simulink model "model"  (R2024b)
settings: Solver=ode45  StartTime=0.0  StopTime=100  RelTol=1e-3
undefined symbols (not defined in the file or in its folder): X, Y, Z
libraries: sm_lib x36, robotlib x19, nesl_utility x9, slpidlib x4, sharedtransform x1
settings Model: Creator=tmood  LastModifiedBy=tmood

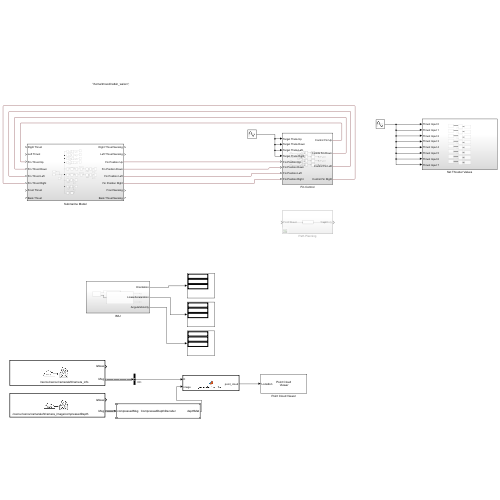
[thumbnail: Simulink's stored preview of the top-level diagram]
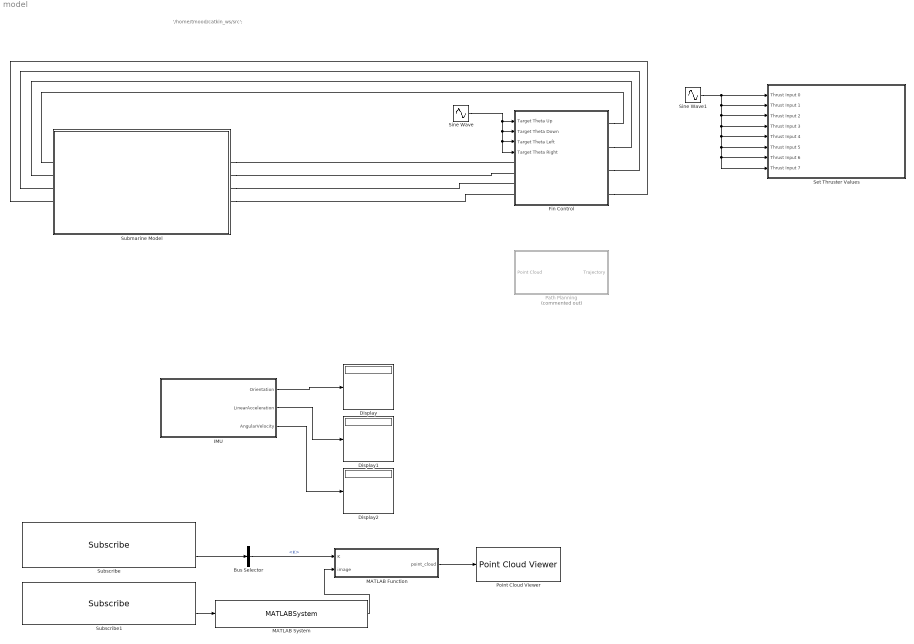
== system model ==
  note: '/home/tmood/catkin_ws/src';
  Bus Selector : BusSelector  OutputSignals=K
  Display : Display
  Display1 : Display
  Display2 : Display
  Fin Control : Subsystem
  IMU : Subsystem
  MATLAB Function : MATLAB Function  TreatAsAtomicUnit=on
  MATLAB System : MATLABSystem  System=CompressedDepthDecoder  SimulateUsing=Interpreted execution
      mask Type: CompressedDepthDecoder
      mask Display:
      | disp('CompressedDepthDecoder');
      | port_label('input',1,'compressedMsg');
      | port_label('output',1,'depthMat');
  Path Planning : Subsystem  Commented=on
  Point Cloud Viewer : PointCloudViewer  FigPos=[665.8 703.6 409.6 300]
  Set Thruster Values : Subsystem
  Sine Wave : Sin  Amplitude=pi/2  SampleTime=0
  Sine Wave1 : Sin  Amplitude=2000  Frequency=0.1  SampleTime=0
  Submarine Model : Subsystem
  Subscribe : robotlib/Subscribe  topicSource=Select from ROS network  topic=/rexrov/rexrov/cameraleft/camera_info  messageType=sensor_msgs/CameraInfo  SampleTime=-1  legacyBusStruct=off  messageQueueLength=1
  Subscribe1 : robotlib/Subscribe  topicSource=Select from ROS network  topic=/rexrov/rexrov/cameraleft/camera_image/compressedDepth  messageType=sensor_msgs/CompressedImage  SampleTime=-1  legacyBusStruct=off  messageQueueLength=1
  wires:
  Sine Wave/1 -> Fin Control/4(Target Theta Right), Fin Control/3(Target Theta Left), Fin Control/2(Target Theta Down), Fin Control/1(Target Theta Up)
  Sine Wave1/1 -> Set Thruster Values/8(Thrust Input 7), Set Thruster Values/7(Thrust Input 6), Set Thruster Values/6(Thrust Input 5), Set Thruster Values/5(Thrust Input 4), Set Thruster Values/4(Thrust Input 3), Set Thruster Values/3(Thrust Input 2), Set Thruster Values/2(Thrust Input 1), Set Thruster Values/1(Thrust Input 0)
  IMU/1(Orientation) -> Display/1
  IMU/2(LinearAcceleration) -> Display1/1
  IMU/3(AngularVelocity) -> Display2/1
  Subscribe/2 -> Bus Selector/1
  Subscribe1/2 -> MATLAB System/1
  MATLAB Function/1(point_cloud) -> Point Cloud Viewer/1
  Bus Selector/1 -> MATLAB Function/1(K)  "<K>"
  MATLAB System/1 -> MATLAB Function/2(image)
  connections:
  Submarine Model/RConn3 -- Fin Control/LConn1
  Submarine Model/RConn4 -- Fin Control/LConn2
  Submarine Model/RConn5 -- Fin Control/LConn3
  Submarine Model/RConn6 -- Fin Control/LConn4
  Fin Control/RConn1 -- Submarine Model/LConn3
  Fin Control/RConn2 -- Submarine Model/LConn4
  Fin Control/RConn3 -- Submarine Model/LConn5
  Fin Control/RConn4 -- Submarine Model/LConn6

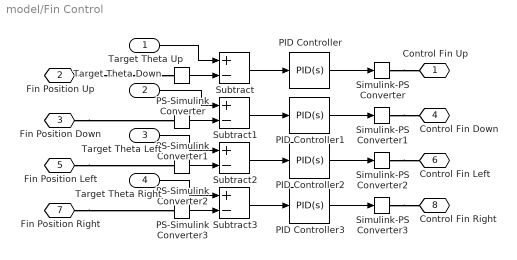
== system model/Fin Control ==
  Target Theta Up : Inport
  Target Theta Down : Inport  Port=2
  Target Theta Left : Inport  Port=3
  Target Theta Right : Inport  Port=4
  PID Controller{,1..3} (4 alike) : slpidlib/PID Controller  Controller=PID  Form=Parallel  TimeDomain=Continuous-time  UseExternalTs=off  SampleTime=-1  IntegratorMethod=Forward Euler  FilterMethod=Forward Euler  ControllerParametersSource=internal  P=1.4  I=0.5  UseKiTs=off  D=1.4  UseExternalDerivativeSource=off  N=100  UseFilter=on  TunerSelectOption=Transfer Function Based (PID Tuner App)  InitialConditionSource=internal  InitialConditionForIntegrator=0.1  InitialConditionForFilter=0  DifferentiatorICPrevScaledInput=0  ExternalReset=none  TrackingMode=off  Kt=1  LimitOutput=off  SatLimitsSource=internal  UpperSaturationLimit=inf  LowerSaturationLimit=-inf  LinearizeAsGain=on  AntiWindupMode=none  Kb=1  LimitIntegrator=off  UpperIntegratorSaturationLimit=inf  LowerIntegratorSaturationLimit=-inf  POutMin=[]  POutMax=[]  IOutMin=[]  IOutMax=[]  DOutMin=[]  DOutMax=[]  NOutMin=[]  NOutMax=[]  SumOutMin=[]  SumOutMax=[]  SaturationOutMin=[]  SaturationOutMax=[]  PParamMin=[]  PParamMax=[]  IParamMin=[]  IParamMax=[]  DParamMin=[]  DParamMax=[]  NParamMin=[]  NParamMax=[]  KbParamMin=[]  KbParamMax=[]  KtParamMin=[]  KtParamMax=[]  KbOutMin=[]  KbOutMax=[]  KtOutMin=[]  KtOutMax=[]  IntegratorOutMin=[]  IntegratorOutMax=[]  FilterOutMin=[]  FilterOutMax=[]  SumI1OutMin=[]  SumI1OutMax=[]  SumI2OutMin=[]  SumI2OutMax=[]  SumI3OutMin=[]  SumI3OutMax=[]  SumI4OutMin=[]  SumI4OutMax=[]  SumDOutMin=[]  SumDOutMax=[]  DifferentiatorOutMin=[]  DifferentiatorOutMax=[]  FilterDiffOutCoefMin=[]  FilterDiffOutCoefMax=[]  ReciprocalOutMin=[]  ReciprocalOutMax=[]  SumDenOutMin=[]  SumDenOutMax=[]  SumNumOutMin=[]  SumNumOutMax=[]  DivideOutMin=[]  DivideOutMax=[]  UdiffTsProdOutMin=[]  UdiffTsProdOutMax=[]  NTsProdOutMin=[]  NTsProdOutMax=[]  UintegralTsProdOutMin=[]  UintegralTsProdOutMax=[]  UngainTsProdOutMin=[]  UngainTsProdOutMax=[]  ClampingZeroOutDataTypeStr=Inherit: Inherit via back propagation  ClampingZeroOutMin=[]  ClampingZeroOutMax=[]  FilterDenConstantOutDataTypeStr=Inherit: Inherit via back propagation  FilterDenConstantOutMin=[]  FilterDenConstantOutMax=[]  PCopyOutDataTypeStr=Inherit: Inherit via back propagation  PCopyOutMin=[]  PCopyOutMax=[]  NCopyOutDataTypeStr=Inherit: Inherit via back propagation  NCopyOutMin=[]  NCopyOutMax=[]  IntegratorContinuousStateAttributes=''  IntegratorStateMustResolveToSignalObject=off  IntegratorRTWStateStorageClass=Auto  FilterContinuousStateAttributes=''  FilterStateMustResolveToSignalObject=off  FilterRTWStateStorageClass=Auto  ParallelPVariant=InternalParameters  IdealPVariant=Disabled  IVariant=InternalParameters  DVariant=InternalParameters  IntegratorVariant=Continuous  SatVariant=Disabled  AWVariant=Passthrough  PCopyVariant=Disabled  TRVariant=Disabled  FdbkBlocksVariant=Forward  IdealPFdbkVariant=Disabled  SatFdbkVariant=Disabled  DerivativeFilterVariant=ContFilter  NVariant=InternalParameters  NCopyVariant=Disabled  FilterICVariant=InternalICsFilter  IntegratorICVariant=InternalICs  ExternalResetVariant=Disabled  TRSumVariant=Passthrough  SumFdbkVariant=Disabled  SumVariant=Sum_PID  TsampFilterVariant=InternalTs  TsampNgainVariant=Passthrough  TsampIntegralVariant=Disabled_SignalSpec  ExternalSaturationOutDataTypeStr=Inherit: Same as second input  DerivativeSourceVariant=ErrorSignal  PreIntVariant=InternalPreInt
  PS-Simulink Converter{,1..3} (4 alike) : nesl_utility/PS-Simulink Converter  PhysicalDomain=network_engine_domain  SubClassName=ps_output  LeftPortType=input  RightPortType=output  PseudoPeriodic=off  Frequencies=[]  VectorFormat=inherit  Unit=inherit  AffineConversion=off
  Simulink-PS Converter{,1..3} (4 alike) : nesl_utility/Simulink-PS Converter  PhysicalDomain=network_engine_domain  SubClassName=ps_input  LeftPortType=input  RightPortType=output  PseudoPeriodic=off  Frequencies=[]  NoiseDistribution=none  NoiseParameters=[]  Unit=1  AffineConversion=off  FilteringAndDerivatives=provide  SimscapeFilterOrder=1  InputFilterTimeConstant=0.001  UdotUserProvided=0
  Subtract{,1..3} (4 alike) : Sum  Inputs=+-
  Control Fin Up : PMIOPort  Side=Right
  Fin Position Up : PMIOPort  Port=2  Side=Left
  Fin Position Down : PMIOPort  Port=3  Side=Left
  Control Fin Down : PMIOPort  Port=4  Side=Right
  Fin Position Left : PMIOPort  Port=5  Side=Left
  Control Fin Left : PMIOPort  Port=6  Side=Right
  Fin Position Right : PMIOPort  Port=7  Side=Left
  Control Fin Right : PMIOPort  Port=8  Side=Right
  wires:
  PID Controller1/1 -> Simulink-PS Converter1/1
  PS-Simulink Converter2/1 -> Subtract2/2
  Target Theta Up/1 -> Subtract/1
  PID Controller2/1 -> Simulink-PS Converter2/1
  PS-Simulink Converter3/1 -> Subtract3/2
  PID Controller/1 -> Simulink-PS Converter/1
  PID Controller3/1 -> Simulink-PS Converter3/1
  Subtract1/1 -> PID Controller1/1
  PS-Simulink Converter1/1 -> Subtract1/2
  Target Theta Down/1 -> Subtract1/1
  PS-Simulink Converter/1 -> Subtract/2
  Target Theta Right/1 -> Subtract3/1
  Subtract/1 -> PID Controller/1
  Subtract2/1 -> PID Controller2/1
  Subtract3/1 -> PID Controller3/1
  Target Theta Left/1 -> Subtract2/1
  connections:
  Fin Position Down/RConn1 -- PS-Simulink Converter1/LConn1
  Simulink-PS Converter2/RConn1 -- Control Fin Left/RConn1
  Simulink-PS Converter/RConn1 -- Control Fin Up/RConn1
  Fin Position Left/RConn1 -- PS-Simulink Converter2/LConn1
  Simulink-PS Converter1/RConn1 -- Control Fin Down/RConn1
  Fin Position Right/RConn1 -- PS-Simulink Converter3/LConn1
  Fin Position Up/RConn1 -- PS-Simulink Converter/LConn1
  Simulink-PS Converter3/RConn1 -- Control Fin Right/RConn1

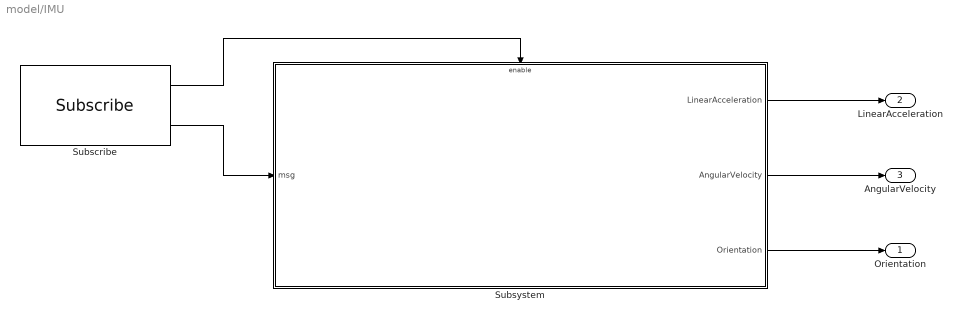
== system model/IMU ==
  Subscribe : robotlib/Subscribe  topicSource=Select from ROS network  topic=/rexrov/imu  messageType=sensor_msgs/Imu  SampleTime=-1  legacyBusStruct=off  messageQueueLength=1
  Subsystem : Subsystem
  Orientation : Outport
  LinearAcceleration : Outport  Port=2
  AngularVelocity : Outport  Port=3
  wires:
  Subscribe/2 -> Subsystem/1(msg)
  Subsystem/1(LinearAcceleration) -> LinearAcceleration/1
  Subsystem/2(AngularVelocity) -> AngularVelocity/1
  Subsystem/3(Orientation) -> Orientation/1
  Subscribe/1 -> Subsystem/Enable

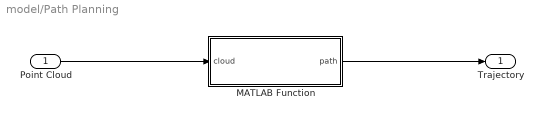
== system model/Path Planning ==
  Point Cloud : Inport
  MATLAB Function : MATLAB Function  TreatAsAtomicUnit=on
  Trajectory : Outport
  wires:
  Point Cloud/1 -> MATLAB Function/1(cloud)
  MATLAB Function/1(path) -> Trajectory/1

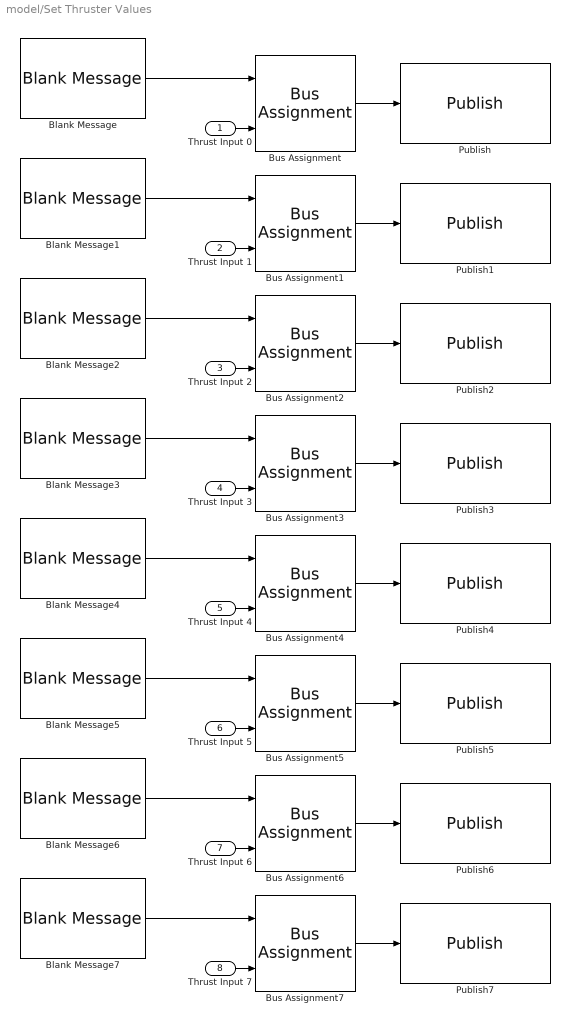
== system model/Set Thruster Values ==
  Thrust Input 0 : Inport
  Thrust Input 1 : Inport  Port=2
  Thrust Input 2 : Inport  Port=3
  Thrust Input 3 : Inport  Port=4
  Thrust Input 4 : Inport  Port=5
  Thrust Input 5 : Inport  Port=6
  Thrust Input 6 : Inport  Port=7
  Thrust Input 7 : Inport  Port=8
  Blank Message{,1..7} (8 alike) : robotlib/Blank Message  messageClass=Message  entityType=uuv_gazebo_ros_plugins_msgs/FloatStamped  messageType=uuv_gazebo_ros_plugins_msgs/FloatStamped  SampleTime=inf  legacyBusStruct=off
  Bus Assignment{,1..7} (8 alike) : BusAssignment  AssignedSignals=Data
  Publish : robotlib/Publish  topicSource=Select from ROS network  topic=/rexrov/thrusters/0/input  messageType=uuv_gazebo_ros_plugins_msgs/FloatStamped  legacyBusStruct=off  messageQueueLength=1
  Publish1 : robotlib/Publish  topicSource=Select from ROS network  topic=/rexrov/thrusters/1/input  messageType=uuv_gazebo_ros_plugins_msgs/FloatStamped  legacyBusStruct=off  messageQueueLength=1
  Publish2 : robotlib/Publish  topicSource=Select from ROS network  topic=/rexrov/thrusters/2/input  messageType=uuv_gazebo_ros_plugins_msgs/FloatStamped  legacyBusStruct=off  messageQueueLength=1
  Publish3 : robotlib/Publish  topicSource=Select from ROS network  topic=/rexrov/thrusters/3/input  messageType=uuv_gazebo_ros_plugins_msgs/FloatStamped  legacyBusStruct=off  messageQueueLength=1
  Publish4 : robotlib/Publish  topicSource=Select from ROS network  topic=/rexrov/thrusters/4/input  messageType=uuv_gazebo_ros_plugins_msgs/FloatStamped  legacyBusStruct=off  messageQueueLength=1
  Publish5 : robotlib/Publish  topicSource=Select from ROS network  topic=/rexrov/thrusters/5/input  messageType=uuv_gazebo_ros_plugins_msgs/FloatStamped  legacyBusStruct=off  messageQueueLength=1
  Publish6 : robotlib/Publish  topicSource=Select from ROS network  topic=/rexrov/thrusters/6/input  messageType=uuv_gazebo_ros_plugins_msgs/FloatStamped  legacyBusStruct=off  messageQueueLength=1
  Publish7 : robotlib/Publish  topicSource=Select from ROS network  topic=/rexrov/thrusters/7/input  messageType=uuv_gazebo_ros_plugins_msgs/FloatStamped  legacyBusStruct=off  messageQueueLength=1
  wires:
  Bus Assignment2/1 -> Publish2/1
  Blank Message7/1 -> Bus Assignment7/1
  Thrust Input 3/1 -> Bus Assignment3/2
  Blank Message6/1 -> Bus Assignment6/1
  Thrust Input 1/1 -> Bus Assignment1/2
  Bus Assignment6/1 -> Publish6/1
  Bus Assignment5/1 -> Publish5/1
  Bus Assignment4/1 -> Publish4/1
  Thrust Input 0/1 -> Bus Assignment/2
  Bus Assignment3/1 -> Publish3/1
  Blank Message/1 -> Bus Assignment/1
  Blank Message4/1 -> Bus Assignment4/1
  Blank Message1/1 -> Bus Assignment1/1
  Bus Assignment/1 -> Publish/1
  Bus Assignment1/1 -> Publish1/1
  Blank Message5/1 -> Bus Assignment5/1
  Thrust Input 6/1 -> Bus Assignment6/2
  Blank Message3/1 -> Bus Assignment3/1
  Blank Message2/1 -> Bus Assignment2/1
  Bus Assignment7/1 -> Publish7/1
  Thrust Input 4/1 -> Bus Assignment4/2
  Thrust Input 5/1 -> Bus Assignment5/2
  Thrust Input 2/1 -> Bus Assignment2/2
  Thrust Input 7/1 -> Bus Assignment7/2

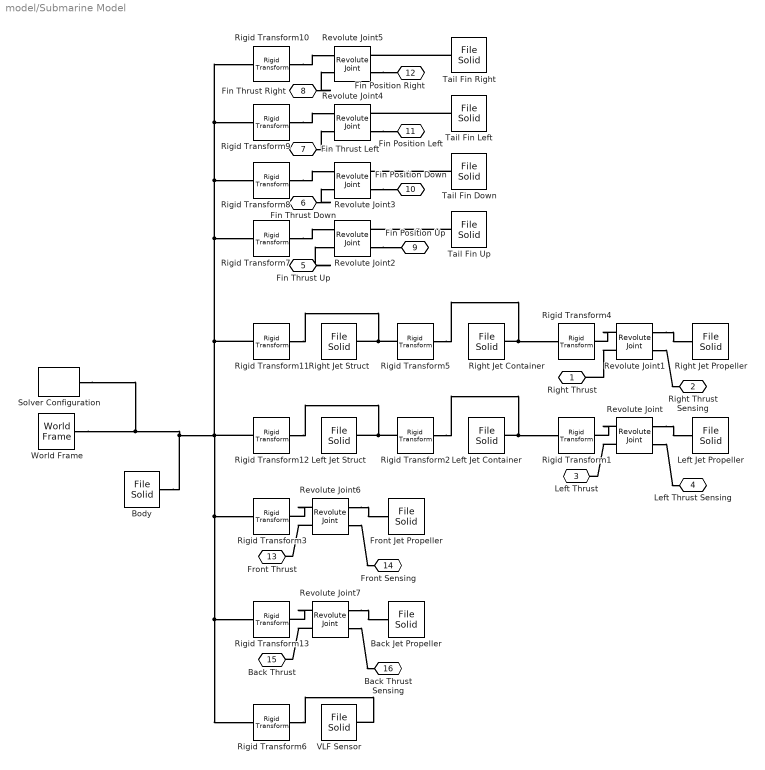
== system model/Submarine Model ==
  Back Jet Propeller : sm_lib/Body Elements/File Solid  ExtGeomFileName=C:\Programming\Competitions\MATLAB\Underwater-Drone\Simulation\Models\jet_turbine.obj  UnitType=Custom  ExtGeomFileUnits=cm  StepReaderType=HEX  ExportConvexHullGeometry=off  InertiaType=CalculateFromGeometry  BasedOnType=Density  Density=DENSITY  DensityUnits=kg/m^3  Mass=1  MassUnits=kg  CenterOfMass=[0 0 0]  CenterOfMassUnits=m  MomentsOfInertia=[1 1 1]  MomentsOfInertiaUnits=kg*m^2  ProductsOfInertia=[0 0 0]  ProductsOfInertiaUnits=kg*m^2  GraphicType=FromGeometry  MarkerShape=Sphere  MarkerSize=10  GraphicVisPropType=SimpleVisualProperties  GraphicDiffuseColor=[0.9 0.9 0.9]  GraphicOpacity=1  GraphicSpecularColor=[0.5 0.5 0.5 1.0]  GraphicAmbientColor=[0.15 0.15 0.15 1.0]  GraphicEmissiveColor=[0.0 0.0 0.0 1.0]  GraphicShininess=75  DoExposeReferenceFrame=on  SerializedFrames=<Frames/>
  Body : sm_lib/Body Elements/File Solid  ExtGeomFileName=C:\Programming\Competitions\MATLAB\Underwater-Drone\Simulation\Models\sub_body.obj  UnitType=Custom  ExtGeomFileUnits=cm  StepReaderType=HEX  ExportConvexHullGeometry=off  InertiaType=CalculateFromGeometry  BasedOnType=Density  Density=DENSITY  DensityUnits=kg/m^3  Mass=1  MassUnits=kg  CenterOfMass=[0 0 0]  CenterOfMassUnits=m  MomentsOfInertia=[1 1 1]  MomentsOfInertiaUnits=kg*m^2  ProductsOfInertia=[0 0 0]  ProductsOfInertiaUnits=kg*m^2  GraphicType=FromGeometry  MarkerShape=Sphere  MarkerSize=10  GraphicVisPropType=SimpleVisualProperties  GraphicDiffuseColor=[0.5 0.5 0.5]  GraphicOpacity=1  GraphicSpecularColor=[0.5 0.5 0.5 1.0]  GraphicAmbientColor=[0.15 0.15 0.15 1.0]  GraphicEmissiveColor=[0.0 0.0 0.0 1.0]  GraphicShininess=75  DoExposeReferenceFrame=on  SerializedFrames=<Frames/>
  Front Jet Propeller : sm_lib/Body Elements/File Solid  ExtGeomFileName=C:\Programming\Competitions\MATLAB\Underwater-Drone\Simulation\Models\jet_turbine.obj  UnitType=Custom  ExtGeomFileUnits=cm  StepReaderType=HEX  ExportConvexHullGeometry=off  InertiaType=CalculateFromGeometry  BasedOnType=Density  Density=DENSITY  DensityUnits=kg/m^3  Mass=1  MassUnits=kg  CenterOfMass=[0 0 0]  CenterOfMassUnits=m  MomentsOfInertia=[1 1 1]  MomentsOfInertiaUnits=kg*m^2  ProductsOfInertia=[0 0 0]  ProductsOfInertiaUnits=kg*m^2  GraphicType=FromGeometry  MarkerShape=Sphere  MarkerSize=10  GraphicVisPropType=SimpleVisualProperties  GraphicDiffuseColor=[0.9 0.9 0.9]  GraphicOpacity=1  GraphicSpecularColor=[0.5 0.5 0.5 1.0]  GraphicAmbientColor=[0.15 0.15 0.15 1.0]  GraphicEmissiveColor=[0.0 0.0 0.0 1.0]  GraphicShininess=75  DoExposeReferenceFrame=on  SerializedFrames=<Frames/>
  Left Jet Container : sm_lib/Body Elements/File Solid  ExtGeomFileName=C:\Programming\Competitions\MATLAB\Underwater-Drone\Simulation\Models\jet_container.obj  UnitType=Custom  ExtGeomFileUnits=mm  StepReaderType=HEX  ExportConvexHullGeometry=off  InertiaType=CalculateFromGeometry  BasedOnType=Density  Density=DENSITY  DensityUnits=kg/m^3  Mass=1  MassUnits=kg  CenterOfMass=[0 0 0]  CenterOfMassUnits=m  MomentsOfInertia=[1 1 1]  MomentsOfInertiaUnits=kg*m^2  ProductsOfInertia=[0 0 0]  ProductsOfInertiaUnits=kg*m^2  GraphicType=FromGeometry  MarkerShape=Sphere  MarkerSize=10  GraphicVisPropType=SimpleVisualProperties  GraphicDiffuseColor=[0.5 0.5 0.5]  GraphicOpacity=1  GraphicSpecularColor=[0.5 0.5 0.5 1.0]  GraphicAmbientColor=[0.15 0.15 0.15 1.0]  GraphicEmissiveColor=[0.0 0.0 0.0 1.0]  GraphicShininess=75  DoExposeReferenceFrame=on  SerializedFrames=<Frames/>
  Left Jet Propeller : sm_lib/Body Elements/File Solid  ExtGeomFileName=C:\Programming\Competitions\MATLAB\Underwater-Drone\Simulation\Models\jet_turbine.obj  UnitType=Custom  ExtGeomFileUnits=cm  StepReaderType=HEX  ExportConvexHullGeometry=off  InertiaType=CalculateFromGeometry  BasedOnType=Density  Density=DENSITY  DensityUnits=kg/m^3  Mass=1  MassUnits=kg  CenterOfMass=[0 0 0]  CenterOfMassUnits=m  MomentsOfInertia=[1 1 1]  MomentsOfInertiaUnits=kg*m^2  ProductsOfInertia=[0 0 0]  ProductsOfInertiaUnits=kg*m^2  GraphicType=FromGeometry  MarkerShape=Sphere  MarkerSize=10  GraphicVisPropType=SimpleVisualProperties  GraphicDiffuseColor=[0.9 0.9 0.9]  GraphicOpacity=1  GraphicSpecularColor=[0.5 0.5 0.5 1.0]  GraphicAmbientColor=[0.15 0.15 0.15 1.0]  GraphicEmissiveColor=[0.0 0.0 0.0 1.0]  GraphicShininess=75  DoExposeReferenceFrame=on  SerializedFrames=<Frames/>
  Left Jet Struct : sm_lib/Body Elements/File Solid  ExtGeomFileName=C:\Programming\Competitions\MATLAB\Underwater-Drone\Simulation\Models\jet_struct.obj  UnitType=Custom  ExtGeomFileUnits=mm  StepReaderType=HEX  ExportConvexHullGeometry=off  InertiaType=CalculateFromGeometry  BasedOnType=Density  Density=DENSITY  DensityUnits=kg/m^3  Mass=1  MassUnits=kg  CenterOfMass=[0 0 0]  CenterOfMassUnits=m  MomentsOfInertia=[1 1 1]  MomentsOfInertiaUnits=kg*m^2  ProductsOfInertia=[0 0 0]  ProductsOfInertiaUnits=kg*m^2  GraphicType=FromGeometry  MarkerShape=Sphere  MarkerSize=10  GraphicVisPropType=SimpleVisualProperties  GraphicDiffuseColor=[0.5 0.5 0.5]  GraphicOpacity=1  GraphicSpecularColor=[0.5 0.5 0.5 1.0]  GraphicAmbientColor=[0.15 0.15 0.15 1.0]  GraphicEmissiveColor=[0.0 0.0 0.0 1.0]  GraphicShininess=75  DoExposeReferenceFrame=on  SerializedFrames=<Frames/>
  Revolute Joint{,1,6..7} (4 alike) : sm_lib/Joints/Revolute Joint  JointMode=Normal  CompositeWrenchDir=FollowerOnBase  CompositeWrenchFrame=BaseFrame  SenseConstraintForce=off  SenseConstraintTorque=off  SenseTotalForce=off  SenseTotalTorque=off  PositionTargetSpecify=off  PositionTargetPriority=High  PositionTargetValue=0  PositionTargetValueUnits=deg  VelocityTargetSpecify=off  VelocityTargetPriority=High  VelocityTargetValue=0  VelocityTargetValueUnits=deg/s  EquilibriumPosition=0  EquilibriumPositionUnits=deg  SpringStiffness=0  SpringStiffnessUnits=N*m/deg  DampingCoefficient=0  DampingCoefficientUnits=N*m/(deg/s)  LowerLimitSpecify=off  LowerLimitBound=-90  LowerLimitBoundUnits=deg  LowerLimitStiffness=1e4  LowerLimitStiffnessUnits=N*m/deg  LowerLimitDamping=10  LowerLimitDampingUnits=N*m/(deg/s)  LowerLimitTransitionRegionWidth=0.1  LowerLimitTransitionRegionWidthUnits=deg  UpperLimitSpecify=off  UpperLimitBound=90  UpperLimitBoundUnits=deg  UpperLimitStiffness=1e4  UpperLimitStiffnessUnits=N*m/deg  UpperLimitDamping=10  UpperLimitDampingUnits=N*m/(deg/s)  UpperLimitTransitionRegionWidth=0.1  UpperLimitTransitionRegionWidthUnits=deg  TorqueActuationMode=InputTorque  MotionActuationMode=ComputedMotion  SensePosition=off  SenseVelocity=off  SenseAcceleration=off  SenseTorqueForce=on  SenseLowerLimitTorqueForce=off  SenseUpperLimitTorqueForce=off
  Revolute Joint{2..5} (4 alike) : sm_lib/Joints/Revolute Joint  JointMode=Normal  CompositeWrenchDir=FollowerOnBase  CompositeWrenchFrame=BaseFrame  SenseConstraintForce=off  SenseConstraintTorque=off  SenseTotalForce=off  SenseTotalTorque=off  PositionTargetSpecify=off  PositionTargetPriority=High  PositionTargetValue=0  PositionTargetValueUnits=deg  VelocityTargetSpecify=off  VelocityTargetPriority=High  VelocityTargetValue=0  VelocityTargetValueUnits=deg/s  EquilibriumPosition=0  EquilibriumPositionUnits=deg  SpringStiffness=0  SpringStiffnessUnits=N*m/deg  DampingCoefficient=0  DampingCoefficientUnits=N*m/(deg/s)  LowerLimitSpecify=off  LowerLimitBound=-90  LowerLimitBoundUnits=deg  LowerLimitStiffness=1e4  LowerLimitStiffnessUnits=N*m/deg  LowerLimitDamping=10  LowerLimitDampingUnits=N*m/(deg/s)  LowerLimitTransitionRegionWidth=0.1  LowerLimitTransitionRegionWidthUnits=deg  UpperLimitSpecify=off  UpperLimitBound=90  UpperLimitBoundUnits=deg  UpperLimitStiffness=1e4  UpperLimitStiffnessUnits=N*m/deg  UpperLimitDamping=10  UpperLimitDampingUnits=N*m/(deg/s)  UpperLimitTransitionRegionWidth=0.1  UpperLimitTransitionRegionWidthUnits=deg  TorqueActuationMode=InputTorque  MotionActuationMode=ComputedMotion  SensePosition=on  SenseVelocity=off  SenseAcceleration=off  SenseTorqueForce=off  SenseLowerLimitTorqueForce=off  SenseUpperLimitTorqueForce=off
  Right Jet Container : sm_lib/Body Elements/File Solid  ExtGeomFileName=C:\Programming\Competitions\MATLAB\Underwater-Drone\Simulation\Models\jet_container.obj  UnitType=Custom  ExtGeomFileUnits=mm  StepReaderType=HEX  ExportConvexHullGeometry=off  InertiaType=CalculateFromGeometry  BasedOnType=Density  Density=DENSITY  DensityUnits=kg/m^3  Mass=1  MassUnits=kg  CenterOfMass=[0 0 0]  CenterOfMassUnits=m  MomentsOfInertia=[1 1 1]  MomentsOfInertiaUnits=kg*m^2  ProductsOfInertia=[0 0 0]  ProductsOfInertiaUnits=kg*m^2  GraphicType=FromGeometry  MarkerShape=Sphere  MarkerSize=10  GraphicVisPropType=SimpleVisualProperties  GraphicDiffuseColor=[0.5 0.5 0.5]  GraphicOpacity=1  GraphicSpecularColor=[0.5 0.5 0.5 1.0]  GraphicAmbientColor=[0.15 0.15 0.15 1.0]  GraphicEmissiveColor=[0.0 0.0 0.0 1.0]  GraphicShininess=75  DoExposeReferenceFrame=on  SerializedFrames=<Frames/>
  Right Jet Propeller : sm_lib/Body Elements/File Solid  ExtGeomFileName=C:\Programming\Competitions\MATLAB\Underwater-Drone\Simulation\Models\jet_turbine.obj  UnitType=Custom  ExtGeomFileUnits=cm  StepReaderType=HEX  ExportConvexHullGeometry=off  InertiaType=CalculateFromGeometry  BasedOnType=Density  Density=DENSITY  DensityUnits=kg/m^3  Mass=1  MassUnits=kg  CenterOfMass=[0 0 0]  CenterOfMassUnits=m  MomentsOfInertia=[1 1 1]  MomentsOfInertiaUnits=kg*m^2  ProductsOfInertia=[0 0 0]  ProductsOfInertiaUnits=kg*m^2  GraphicType=FromGeometry  MarkerShape=Sphere  MarkerSize=10  GraphicVisPropType=SimpleVisualProperties  GraphicDiffuseColor=[0.9 0.9 0.9]  GraphicOpacity=1  GraphicSpecularColor=[0.5 0.5 0.5 1.0]  GraphicAmbientColor=[0.15 0.15 0.15 1.0]  GraphicEmissiveColor=[0.0 0.0 0.0 1.0]  GraphicShininess=75  DoExposeReferenceFrame=on  SerializedFrames=<Frames/>
  Right Jet Struct : sm_lib/Body Elements/File Solid  ExtGeomFileName=C:\Programming\Competitions\MATLAB\Underwater-Drone\Simulation\Models\jet_struct.obj  UnitType=Custom  ExtGeomFileUnits=mm  StepReaderType=HEX  ExportConvexHullGeometry=off  InertiaType=CalculateFromGeometry  BasedOnType=Density  Density=DENSITY  DensityUnits=kg/m^3  Mass=1  MassUnits=kg  CenterOfMass=[0 0 0]  CenterOfMassUnits=m  MomentsOfInertia=[1 1 1]  MomentsOfInertiaUnits=kg*m^2  ProductsOfInertia=[0 0 0]  ProductsOfInertiaUnits=kg*m^2  GraphicType=FromGeometry  MarkerShape=Sphere  MarkerSize=10  GraphicVisPropType=SimpleVisualProperties  GraphicDiffuseColor=[0.5 0.5 0.5]  GraphicOpacity=1  GraphicSpecularColor=[0.5 0.5 0.5 1.0]  GraphicAmbientColor=[0.15 0.15 0.15 1.0]  GraphicEmissiveColor=[0.0 0.0 0.0 1.0]  GraphicShininess=75  DoExposeReferenceFrame=on  SerializedFrames=<Frames/>
  Rigid Transform1 : sm_lib/Frames and Transforms/Rigid Transform  RotationMethod=RotationSequence  FollAlignAxisA=+X  BaseAlignAxisA=+Y  FollAlignAxisB=+Y  BaseAlignAxisB=+Z  RotationStandardAxis=+Z  RotationAngle=0  RotationAngleUnits=deg  RotationArbitraryAxis=[0 0 1]  RotationSequenceAxes=BaseAxes  RotationSequence=XYZ  RotationSequenceAngles=[-90 0 0]  RotationSequenceAnglesUnits=deg  RotationMatrix=[1 0 0;0 1 0;0 0 1]  Quaternion=[1 0 0 0]  TranslationMethod=Cartesian  TranslationCartesianOffset=[0 0.85 0]  TranslationCartesianOffsetUnits=m  TranslationStandardAxis=+Z  TranslationStandardOffset=0  TranslationStandardOffsetUnits=m  TranslationROffset=0  TranslationROffsetUnits=m  TranslationThetaOffset=0  TranslationThetaOffsetUnits=deg  TranslationZOffset=0  TranslationZOffsetUnits=m
  Rigid Transform10 : sm_lib/Frames and Transforms/Rigid Transform  RotationMethod=RotationSequence  FollAlignAxisA=+X  BaseAlignAxisA=+Y  FollAlignAxisB=+Y  BaseAlignAxisB=+Z  RotationStandardAxis=+Z  RotationAngle=90  RotationAngleUnits=deg  RotationArbitraryAxis=[0 0 1]  RotationSequenceAxes=BaseAxes  RotationSequence=XYZ  RotationSequenceAngles=[-90 0 0]  RotationSequenceAnglesUnits=deg  RotationMatrix=[1 0 0;0 1 0;0 0 1]  Quaternion=[1 0 0 0]  TranslationMethod=Cartesian  TranslationCartesianOffset=[1.8 0.35 0]  TranslationCartesianOffsetUnits=m  TranslationStandardAxis=+Y  TranslationStandardOffset=100  TranslationStandardOffsetUnits=m  TranslationROffset=0  TranslationROffsetUnits=m  TranslationThetaOffset=0  TranslationThetaOffsetUnits=deg  TranslationZOffset=0  TranslationZOffsetUnits=m
  Rigid Transform11 : sm_lib/Frames and Transforms/Rigid Transform  RotationMethod=RotationSequence  FollAlignAxisA=+X  BaseAlignAxisA=+Y  FollAlignAxisB=+Y  BaseAlignAxisB=+Z  RotationStandardAxis=+Z  RotationAngle=0  RotationAngleUnits=deg  RotationArbitraryAxis=[0 0 1]  RotationSequenceAxes=BaseAxes  RotationSequence=XYZ  RotationSequenceAngles=[0 0 90]  RotationSequenceAnglesUnits=deg  RotationMatrix=[1 0 0;0 1 0;0 0 1]  Quaternion=[1 0 0 0]  TranslationMethod=Cartesian  TranslationCartesianOffset=[1.5 0.7 0]  TranslationCartesianOffsetUnits=m  TranslationStandardAxis=+Z  TranslationStandardOffset=0  TranslationStandardOffsetUnits=m  TranslationROffset=0  TranslationROffsetUnits=m  TranslationThetaOffset=0  TranslationThetaOffsetUnits=deg  TranslationZOffset=0  TranslationZOffsetUnits=m
  Rigid Transform12 : sm_lib/Frames and Transforms/Rigid Transform  RotationMethod=RotationSequence  FollAlignAxisA=+X  BaseAlignAxisA=+Y  FollAlignAxisB=+Y  BaseAlignAxisB=+Z  RotationStandardAxis=+Z  RotationAngle=90  RotationAngleUnits=deg  RotationArbitraryAxis=[0 0 1]  RotationSequenceAxes=BaseAxes  RotationSequence=XYZ  RotationSequenceAngles=[0 180 90]  RotationSequenceAnglesUnits=deg  RotationMatrix=[1 0 0;0 1 0;0 0 1]  Quaternion=[1 0 0 0]  TranslationMethod=Cartesian  TranslationCartesianOffset=[1.5 -0.7 0]  TranslationCartesianOffsetUnits=m  TranslationStandardAxis=+Y  TranslationStandardOffset=100  TranslationStandardOffsetUnits=m  TranslationROffset=0  TranslationROffsetUnits=m  TranslationThetaOffset=0  TranslationThetaOffsetUnits=deg  TranslationZOffset=0  TranslationZOffsetUnits=m
  Rigid Transform13 : sm_lib/Frames and Transforms/Rigid Transform  RotationMethod=RotationSequence  FollAlignAxisA=+X  BaseAlignAxisA=+Y  FollAlignAxisB=+Y  BaseAlignAxisB=+Z  RotationStandardAxis=+Z  RotationAngle=0  RotationAngleUnits=deg  RotationArbitraryAxis=[0 0 1]  RotationSequenceAxes=BaseAxes  RotationSequence=XYZ  RotationSequenceAngles=[0 0 0]  RotationSequenceAnglesUnits=deg  RotationMatrix=[1 0 0;0 1 0;0 0 1]  Quaternion=[1 0 0 0]  TranslationMethod=Cartesian  TranslationCartesianOffset=[1.2 0 0.35]  TranslationCartesianOffsetUnits=m  TranslationStandardAxis=+Z  TranslationStandardOffset=0  TranslationStandardOffsetUnits=m  TranslationROffset=0  TranslationROffsetUnits=m  TranslationThetaOffset=0  TranslationThetaOffsetUnits=deg  TranslationZOffset=0  TranslationZOffsetUnits=m
  Rigid Transform2 : sm_lib/Frames and Transforms/Rigid Transform  RotationMethod=None  FollAlignAxisA=+X  BaseAlignAxisA=+Y  FollAlignAxisB=+Y  BaseAlignAxisB=+Z  RotationStandardAxis=+Z  RotationAngle=0  RotationAngleUnits=deg  RotationArbitraryAxis=[0 0 1]  RotationSequenceAxes=FollowerAxes  RotationSequence=XYX  RotationSequenceAngles=[0 0 0]  RotationSequenceAnglesUnits=deg  RotationMatrix=[1 0 0;0 1 0;0 0 1]  Quaternion=[1 0 0 0]  TranslationMethod=None  TranslationCartesianOffset=[0 0 0]  TranslationCartesianOffsetUnits=m  TranslationStandardAxis=+Z  TranslationStandardOffset=0  TranslationStandardOffsetUnits=m  TranslationROffset=0  TranslationROffsetUnits=m  TranslationThetaOffset=0  TranslationThetaOffsetUnits=deg  TranslationZOffset=0  TranslationZOffsetUnits=m
  Rigid Transform3 : sm_lib/Frames and Transforms/Rigid Transform  RotationMethod=RotationSequence  FollAlignAxisA=+X  BaseAlignAxisA=+Y  FollAlignAxisB=+Y  BaseAlignAxisB=+Z  RotationStandardAxis=+Z  RotationAngle=0  RotationAngleUnits=deg  RotationArbitraryAxis=[0 0 1]  RotationSequenceAxes=BaseAxes  RotationSequence=XYZ  RotationSequenceAngles=[0 0 0]  RotationSequenceAnglesUnits=deg  RotationMatrix=[1 0 0;0 1 0;0 0 1]  Quaternion=[1 0 0 0]  TranslationMethod=Cartesian  TranslationCartesianOffset=[0.5 0 0.35]  TranslationCartesianOffsetUnits=m  TranslationStandardAxis=+Z  TranslationStandardOffset=0  TranslationStandardOffsetUnits=m  TranslationROffset=0  TranslationROffsetUnits=m  TranslationThetaOffset=0  TranslationThetaOffsetUnits=deg  TranslationZOffset=0  TranslationZOffsetUnits=m
  Rigid Transform4 : sm_lib/Frames and Transforms/Rigid Transform  RotationMethod=RotationSequence  FollAlignAxisA=+X  BaseAlignAxisA=+Y  FollAlignAxisB=+Y  BaseAlignAxisB=+Z  RotationStandardAxis=+Z  RotationAngle=0  RotationAngleUnits=deg  RotationArbitraryAxis=[0 0 1]  RotationSequenceAxes=FollowerAxes  RotationSequence=XYZ  RotationSequenceAngles=[-90 0 0]  RotationSequenceAnglesUnits=deg  RotationMatrix=[1 0 0;0 1 0;0 0 1]  Quaternion=[1 0 0 0]  TranslationMethod=Cartesian  TranslationCartesianOffset=[0 0.85 0]  TranslationCartesianOffsetUnits=m  TranslationStandardAxis=+Z  TranslationStandardOffset=0  TranslationStandardOffsetUnits=m  TranslationROffset=0  TranslationROffsetUnits=m  TranslationThetaOffset=0  TranslationThetaOffsetUnits=deg  TranslationZOffset=0  TranslationZOffsetUnits=m
  Rigid Transform5 : sm_lib/Frames and Transforms/Rigid Transform  RotationMethod=None  FollAlignAxisA=+X  BaseAlignAxisA=+Y  FollAlignAxisB=+Y  BaseAlignAxisB=+Z  RotationStandardAxis=+Z  RotationAngle=0  RotationAngleUnits=deg  RotationArbitraryAxis=[0 0 1]  RotationSequenceAxes=FollowerAxes  RotationSequence=XYX  RotationSequenceAngles=[0 0 0]  RotationSequenceAnglesUnits=deg  RotationMatrix=[1 0 0;0 1 0;0 0 1]  Quaternion=[1 0 0 0]  TranslationMethod=None  TranslationCartesianOffset=[0 0 0]  TranslationCartesianOffsetUnits=m  TranslationStandardAxis=+Z  TranslationStandardOffset=0  TranslationStandardOffsetUnits=m  TranslationROffset=0  TranslationROffsetUnits=m  TranslationThetaOffset=0  TranslationThetaOffsetUnits=deg  TranslationZOffset=0  TranslationZOffsetUnits=m
  Rigid Transform6 : sm_lib/Frames and Transforms/Rigid Transform  RotationMethod=RotationSequence  FollAlignAxisA=+X  BaseAlignAxisA=+Y  FollAlignAxisB=+Y  BaseAlignAxisB=+Z  RotationStandardAxis=+Z  RotationAngle=0  RotationAngleUnits=deg  RotationArbitraryAxis=[0 0 1]  RotationSequenceAxes=BaseAxes  RotationSequence=XYZ  RotationSequenceAngles=[0 90 0]  RotationSequenceAnglesUnits=deg  RotationMatrix=[1 0 0;0 1 0;0 0 1]  Quaternion=[1 0 0 0]  TranslationMethod=Cartesian  TranslationCartesianOffset=[-0.05 0 0]  TranslationCartesianOffsetUnits=m  TranslationStandardAxis=+Z  TranslationStandardOffset=0  TranslationStandardOffsetUnits=m  TranslationROffset=0  TranslationROffsetUnits=m  TranslationThetaOffset=0  TranslationThetaOffsetUnits=deg  TranslationZOffset=0  TranslationZOffsetUnits=m
  Rigid Transform7 : sm_lib/Frames and Transforms/Rigid Transform  RotationMethod=RotationSequence  FollAlignAxisA=+X  BaseAlignAxisA=+Y  FollAlignAxisB=+Y  BaseAlignAxisB=+Z  RotationStandardAxis=+Z  RotationAngle=90  RotationAngleUnits=deg  RotationArbitraryAxis=[0 0 1]  RotationSequenceAxes=BaseAxes  RotationSequence=XYZ  RotationSequenceAngles=[0 0 0]  RotationSequenceAnglesUnits=deg  RotationMatrix=[1 0 0;0 1 0;0 0 1]  Quaternion=[1 0 0 0]  TranslationMethod=Cartesian  TranslationCartesianOffset=[1.8 0 0.3]  TranslationCartesianOffsetUnits=m  TranslationStandardAxis=+Y  TranslationStandardOffset=100  TranslationStandardOffsetUnits=m  TranslationROffset=0  TranslationROffsetUnits=m  TranslationThetaOffset=0  TranslationThetaOffsetUnits=deg  TranslationZOffset=0  TranslationZOffsetUnits=m
  Rigid Transform8 : sm_lib/Frames and Transforms/Rigid Transform  RotationMethod=RotationSequence  FollAlignAxisA=+X  BaseAlignAxisA=+Y  FollAlignAxisB=+Y  BaseAlignAxisB=+Z  RotationStandardAxis=+Z  RotationAngle=90  RotationAngleUnits=deg  RotationArbitraryAxis=[0 0 1]  RotationSequenceAxes=BaseAxes  RotationSequence=XYZ  RotationSequenceAngles=[180 0 0]  RotationSequenceAnglesUnits=deg  RotationMatrix=[1 0 0;0 1 0;0 0 1]  Quaternion=[1 0 0 0]  TranslationMethod=Cartesian  TranslationCartesianOffset=[1.8 0 -0.3]  TranslationCartesianOffsetUnits=m  TranslationStandardAxis=+Y  TranslationStandardOffset=100  TranslationStandardOffsetUnits=m  TranslationROffset=0  TranslationROffsetUnits=m  TranslationThetaOffset=0  TranslationThetaOffsetUnits=deg  TranslationZOffset=0  TranslationZOffsetUnits=m
  Rigid Transform9 : sm_lib/Frames and Transforms/Rigid Transform  RotationMethod=RotationSequence  FollAlignAxisA=+X  BaseAlignAxisA=+Y  FollAlignAxisB=+Y  BaseAlignAxisB=+Z  RotationStandardAxis=+Z  RotationAngle=90  RotationAngleUnits=deg  RotationArbitraryAxis=[0 0 1]  RotationSequenceAxes=BaseAxes  RotationSequence=XYZ  RotationSequenceAngles=[90 0 0]  RotationSequenceAnglesUnits=deg  RotationMatrix=[1 0 0;0 1 0;0 0 1]  Quaternion=[1 0 0 0]  TranslationMethod=Cartesian  TranslationCartesianOffset=[1.8 -0.35 0]  TranslationCartesianOffsetUnits=m  TranslationStandardAxis=+Y  TranslationStandardOffset=100  TranslationStandardOffsetUnits=m  TranslationROffset=0  TranslationROffsetUnits=m  TranslationThetaOffset=0  TranslationThetaOffsetUnits=deg  TranslationZOffset=0  TranslationZOffsetUnits=m
  Solver Configuration : nesl_utility/Solver Configuration  PhysicalDomain=network_engine_domain  SubClassName=solver  LeftPortType=input  RightPortType=generic  Tones=[]  Harmonics=[]  SimulateNoise=off  Profile=off  UseLocalSampling=off  EnableSwitchedLinearOptims=on  FrequencyDomain=off  UseCCode=off  RelTol=0.001  AbsTol=0.001  MinStep=1e-09  ToWorkspace=off  RevertToSquareIcSolve=off  NumHomotopyIterations=100  PhasorMode=off  PhasorModeNumHarmonics=1  ConsistencySolver=NEWTON_XTOL_AFTER_FTOL  IndexReductionMethod=DerivativeReplacement  DoDC=off  ResidualTolerance=1e-09  ConsistencyTolSource=GLOBAL  ConsistencyAbsTol=0.001  ConsistencyRelTol=0.001  ConsistencyTolFactor=0.001  UseLocalSolver=off  LocalSolverChoice=NE_BACKWARD_EULER_ADVANCER  ResolveIndetEquations=on  FunctionEvalNumThread=1  LocalSolverSampleTime=0.001  DoFixedCost=off  MaxNonlinIter=3  MaxModeIter=2  ComputeImpulses=off  ImpulseIterations=2  LinearAlgebra=auto  LinearAlgebraNumThread=0  EquationFormulation=NE_TIME_EF  DelaysMemoryBudget=1024  AutomaticFiltering=on  FilteringTimeConstant=0.001  PartitionStorageMethod=AS_NEEDED  PartitionMemoryBudget=1024  PartitionMethod=ROBUST  MultibodyUseLocalSolver=off  MultibodyLocalSolverChoice=ODE1  MultibodyLocalSolverSampleTime=0.001
  Tail Fin Down : sm_lib/Body Elements/File Solid  ExtGeomFileName=C:\Programming\Competitions\MATLAB\Underwater-Drone\Simulation\Models\tail_fin.obj  UnitType=Custom  ExtGeomFileUnits=cm  StepReaderType=HEX  ExportConvexHullGeometry=off  InertiaType=CalculateFromGeometry  BasedOnType=Density  Density=DENSITY  DensityUnits=kg/m^3  Mass=1  MassUnits=kg  CenterOfMass=[0 0 0]  CenterOfMassUnits=m  MomentsOfInertia=[1 1 1]  MomentsOfInertiaUnits=kg*m^2  ProductsOfInertia=[0 0 0]  ProductsOfInertiaUnits=kg*m^2  GraphicType=FromGeometry  MarkerShape=Sphere  MarkerSize=10  GraphicVisPropType=SimpleVisualProperties  GraphicDiffuseColor=[0.5 0.5 0.5]  GraphicOpacity=1  GraphicSpecularColor=[0.5 0.5 0.5 1.0]  GraphicAmbientColor=[0.15 0.15 0.15 1.0]  GraphicEmissiveColor=[0.0 0.0 0.0 1.0]  GraphicShininess=75  DoExposeReferenceFrame=on  SerializedFrames=<Frames/>
  Tail Fin Left : sm_lib/Body Elements/File Solid  ExtGeomFileName=C:\Programming\Competitions\MATLAB\Underwater-Drone\Simulation\Models\tail_fin.obj  UnitType=Custom  ExtGeomFileUnits=cm  StepReaderType=HEX  ExportConvexHullGeometry=off  InertiaType=CalculateFromGeometry  BasedOnType=Density  Density=DENSITY  DensityUnits=kg/m^3  Mass=1  MassUnits=kg  CenterOfMass=[0 0 0]  CenterOfMassUnits=m  MomentsOfInertia=[1 1 1]  MomentsOfInertiaUnits=kg*m^2  ProductsOfInertia=[0 0 0]  ProductsOfInertiaUnits=kg*m^2  GraphicType=FromGeometry  MarkerShape=Sphere  MarkerSize=10  GraphicVisPropType=SimpleVisualProperties  GraphicDiffuseColor=[0.5 0.5 0.5]  GraphicOpacity=1  GraphicSpecularColor=[0.5 0.5 0.5 1.0]  GraphicAmbientColor=[0.15 0.15 0.15 1.0]  GraphicEmissiveColor=[0.0 0.0 0.0 1.0]  GraphicShininess=75  DoExposeReferenceFrame=on  SerializedFrames=<Frames/>
  Tail Fin Right : sm_lib/Body Elements/File Solid  ExtGeomFileName=C:\Programming\Competitions\MATLAB\Underwater-Drone\Simulation\Models\tail_fin.obj  UnitType=Custom  ExtGeomFileUnits=cm  StepReaderType=HEX  ExportConvexHullGeometry=off  InertiaType=CalculateFromGeometry  BasedOnType=Density  Density=DENSITY  DensityUnits=kg/m^3  Mass=1  MassUnits=kg  CenterOfMass=[0 0 0]  CenterOfMassUnits=m  MomentsOfInertia=[1 1 1]  MomentsOfInertiaUnits=kg*m^2  ProductsOfInertia=[0 0 0]  ProductsOfInertiaUnits=kg*m^2  GraphicType=FromGeometry  MarkerShape=Sphere  MarkerSize=10  GraphicVisPropType=SimpleVisualProperties  GraphicDiffuseColor=[0.5 0.5 0.5]  GraphicOpacity=1  GraphicSpecularColor=[0.5 0.5 0.5 1.0]  GraphicAmbientColor=[0.15 0.15 0.15 1.0]  GraphicEmissiveColor=[0.0 0.0 0.0 1.0]  GraphicShininess=75  DoExposeReferenceFrame=on  SerializedFrames=<Frames/>
  Tail Fin Up : sm_lib/Body Elements/File Solid  ExtGeomFileName=C:\Programming\Competitions\MATLAB\Underwater-Drone\Simulation\Models\tail_fin.obj  UnitType=Custom  ExtGeomFileUnits=cm  StepReaderType=HEX  ExportConvexHullGeometry=off  InertiaType=CalculateFromGeometry  BasedOnType=Density  Density=DENSITY  DensityUnits=kg/m^3  Mass=1  MassUnits=kg  CenterOfMass=[0 0 0]  CenterOfMassUnits=m  MomentsOfInertia=[1 1 1]  MomentsOfInertiaUnits=kg*m^2  ProductsOfInertia=[0 0 0]  ProductsOfInertiaUnits=kg*m^2  GraphicType=FromGeometry  MarkerShape=Sphere  MarkerSize=10  GraphicVisPropType=SimpleVisualProperties  GraphicDiffuseColor=[0.5 0.5 0.5]  GraphicOpacity=1  GraphicSpecularColor=[0.5 0.5 0.5 1.0]  GraphicAmbientColor=[0.15 0.15 0.15 1.0]  GraphicEmissiveColor=[0.0 0.0 0.0 1.0]  GraphicShininess=75  DoExposeReferenceFrame=on  SerializedFrames=<Frames/>
  VLF Sensor : sm_lib/Body Elements/File Solid  ExtGeomFileName=C:\Programming\Competitions\MATLAB\Underwater-Drone\Simulation\Models\vlf_distance_sensor.obj  UnitType=Custom  ExtGeomFileUnits=mm  StepReaderType=HEX  ExportConvexHullGeometry=off  InertiaType=CalculateFromGeometry  BasedOnType=Density  Density=DENSITY  DensityUnits=kg/m^3  Mass=1  MassUnits=kg  CenterOfMass=[0 0 0]  CenterOfMassUnits=m  MomentsOfInertia=[1 1 1]  MomentsOfInertiaUnits=kg*m^2  ProductsOfInertia=[0 0 0]  ProductsOfInertiaUnits=kg*m^2  GraphicType=FromGeometry  MarkerShape=Sphere  MarkerSize=10  GraphicVisPropType=SimpleVisualProperties  GraphicDiffuseColor=[0.5 0.5 0.5]  GraphicOpacity=1  GraphicSpecularColor=[0.5 0.5 0.5 1.0]  GraphicAmbientColor=[0.15 0.15 0.15 1.0]  GraphicEmissiveColor=[0.0 0.0 0.0 1.0]  GraphicShininess=75  DoExposeReferenceFrame=on  SerializedFrames=<Frames/>
  World Frame : sm_lib/Frames and Transforms/World Frame
  Right Thrust : PMIOPort  Side=Left
  Right Thrust Sensing : PMIOPort  Port=2  Side=Right
  Left Thrust : PMIOPort  Port=3  Side=Left
  Left Thrust Sensing : PMIOPort  Port=4  Side=Right
  Fin Thrust Up : PMIOPort  Port=5  Side=Left
  Fin Thrust Down : PMIOPort  Port=6  Side=Left
  Fin Thrust Left : PMIOPort  Port=7  Side=Left
  Fin Thrust Right : PMIOPort  Port=8  Side=Left
  Fin Position Up : PMIOPort  Port=9  Side=Right
  Fin Position Down : PMIOPort  Port=10  Side=Right
  Fin Position Left : PMIOPort  Port=11  Side=Right
  Fin Position Right : PMIOPort  Port=12  Side=Right
  Front Thrust : PMIOPort  Port=13  Side=Left
  Front Sensing : PMIOPort  Port=14  Side=Right
  Back Thrust : PMIOPort  Port=15  Side=Left
  Back Thrust Sensing : PMIOPort  Port=16  Side=Right
  connections:
  Rigid Transform2/LConn1 -- Rigid Transform12/RConn1 -- Left Jet Struct/RConn1
  Rigid Transform5/LConn1 -- Rigid Transform11/RConn1 -- Right Jet Struct/RConn1
  World Frame/RConn1 -- Body/RConn1 -- Rigid Transform3/LConn1 -- Rigid Transform13/LConn1 -- Rigid Transform6/LConn1 -- Rigid Transform12/LConn1 -- Rigid Transform11/LConn1 -- Rigid Transform9/LConn1 -- Rigid Transform10/LConn1 -- Rigid Transform8/LConn1 -- Rigid Transform7/LConn1 -- Solver Configuration/RConn1
  Right Jet Container/RConn1 -- Rigid Transform5/RConn1 -- Rigid Transform4/LConn1
  Revolute Joint/LConn1 -- Rigid Transform1/RConn1
  Revolute Joint/RConn1 -- Left Jet Propeller/RConn1
  Revolute Joint1/RConn1 -- Right Jet Propeller/RConn1
  Revolute Joint1/LConn1 -- Rigid Transform4/RConn1
  Rigid Transform2/RConn1 -- Rigid Transform1/LConn1 -- Left Jet Container/RConn1
  Rigid Transform6/RConn1 -- VLF Sensor/RConn1
  Revolute Joint/LConn2 -- Left Thrust/RConn1
  Revolute Joint/RConn2 -- Left Thrust Sensing/RConn1
  Revolute Joint1/RConn2 -- Right Thrust Sensing/RConn1
  Revolute Joint1/LConn2 -- Right Thrust/RConn1
  Rigid Transform7/RConn1 -- Revolute Joint2/LConn1
  Tail Fin Up/RConn1 -- Revolute Joint2/RConn1
  Rigid Transform8/RConn1 -- Revolute Joint3/LConn1
  Tail Fin Down/RConn1 -- Revolute Joint3/RConn1
  Rigid Transform9/RConn1 -- Revolute Joint4/LConn1
  Tail Fin Left/RConn1 -- Revolute Joint4/RConn1
  Rigid Transform10/RConn1 -- Revolute Joint5/LConn1
  Tail Fin Right/RConn1 -- Revolute Joint5/RConn1
  Fin Thrust Up/RConn1 -- Revolute Joint2/LConn2
  Fin Thrust Down/RConn1 -- Revolute Joint3/LConn2
  Fin Thrust Left/RConn1 -- Revolute Joint4/LConn2
  Fin Thrust Right/RConn1 -- Revolute Joint5/LConn2
  Revolute Joint2/RConn2 -- Fin Position Up/RConn1
  Revolute Joint3/RConn2 -- Fin Position Down/RConn1
  Revolute Joint4/RConn2 -- Fin Position Left/RConn1
  Revolute Joint5/RConn2 -- Fin Position Right/RConn1
  Revolute Joint6/LConn2 -- Front Thrust/RConn1
  Revolute Joint6/RConn1 -- Front Jet Propeller/RConn1
  Revolute Joint6/LConn1 -- Rigid Transform3/RConn1
  Revolute Joint6/RConn2 -- Front Sensing/RConn1
  Revolute Joint7/LConn2 -- Back Thrust/RConn1
  Revolute Joint7/LConn1 -- Rigid Transform13/RConn1
  Revolute Joint7/RConn1 -- Back Jet Propeller/RConn1
  Revolute Joint7/RConn2 -- Back Thrust Sensing/RConn1

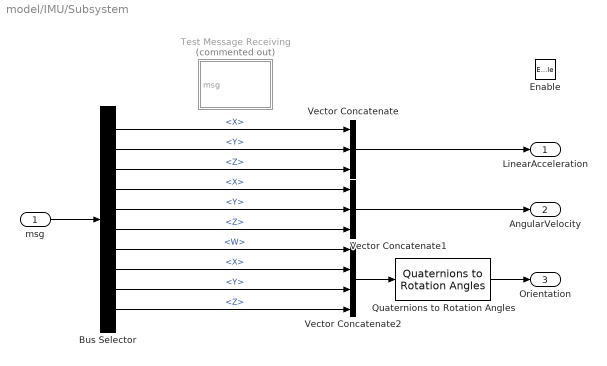
== system model/IMU/Subsystem ==
  msg : Inport
  Enable : EnablePort
  Bus Selector : BusSelector  OutputSignals=LinearAcceleration.X,LinearAcceleration.Y,LinearAcceleration.Z,AngularVelocity.X,AngularVelocity.Y,AngularVelocity.Z,Orientation.W,Orientation.X,Orientation.Y,Orientation.Z
  Quaternions to Rotation Angles : sharedtransform/Quaternions to Rotation Angles  rotationOrder=XYZ  aMode=aMode
  Test Message Receiving : MATLAB Function  Commented=on  TreatAsAtomicUnit=on
  Vector Concatenate : Concatenate  NumInputs=3
  Vector Concatenate1 : Concatenate  NumInputs=3
  Vector Concatenate2 : Concatenate  NumInputs=4
  LinearAcceleration : Outport
  AngularVelocity : Outport  Port=2
  Orientation : Outport  Port=3
  wires:
  Bus Selector/3 -> Vector Concatenate/3  "<Z>"
  Bus Selector/8 -> Vector Concatenate2/2  "<X>"
  Bus Selector/5 -> Vector Concatenate1/2  "<Y>"
  Bus Selector/6 -> Vector Concatenate1/3  "<Z>"
  Bus Selector/7 -> Vector Concatenate2/1  "<W>"
  Bus Selector/2 -> Vector Concatenate/2  "<Y>"
  Bus Selector/4 -> Vector Concatenate1/1  "<X>"
  Quaternions to Rotation Angles/1 -> Orientation/1
  msg/1 -> Bus Selector/1
  Bus Selector/1 -> Vector Concatenate/1  "<X>"
  Bus Selector/9 -> Vector Concatenate2/3  "<Y>"
  Vector Concatenate2/1 -> Quaternions to Rotation Angles/1
  Bus Selector/10 -> Vector Concatenate2/4  "<Z>"
  Vector Concatenate/1 -> LinearAcceleration/1
  Vector Concatenate1/1 -> AngularVelocity/1

== matlab function model/Path Planning/MATLAB Function ==
  data: cloud input; path output
function path = pathPlanning(cloud)
    if isempty(cloud) || (length(cloud) < 1)
        path = NaN;
        return
    end

    pc = pointCloud(cloud); %converts xyz points to MATLAB point cloud

    % cluster_labels = pcsegdist(pc,1); %segments the point cloud, chooses points within 1m
    % 
    % %get the largest cluster
    % counts = histcounts(cluster_labels, 'BinMethod', 'integers');
    % [~, largestCluster] = max(counts);
    % 
    % idx = cluster_labels == largestCluster;

    local_seg = pc.Location(:, :);

    avg_z = mean(local_seg(:,3)); % find the vertical middle of the point cloud
    max_z = max(local_seg(:,3)); %highest point


    % middle_layer = local_seg( (local_seg(:,3) < (avg_z + 1)) && (local_seg(:,3) > (avg_z - 1)) ); %selects all points in the middle of the point cloud with a range of 2m about the average z coord

    middle_layer = local_seg;

    path = middle_layer;
end

== matlab function model/MATLAB Function ==
  data: K input; point_cloud output; image input
function point_cloud = generatePointCloud(K, image)
    fx = K(1);
    fy = K(5);
    cx = K(3);
    cy = K(6);
    
    % Get image size
    [rows, cols] = size(image);
    
    % Create meshgrid of pixel coordinates
    [X, Y] = meshgrid(0:cols-1, 0:rows-1);
    
    % Ensure depth is in double
    Z = double(image);
    X = (X - cx) .* Z / fx;
    Y = (Y - cy) .* Z / fy;
    
    % Output is MxNx3
    point_cloud = cat(3, X, Y, Z);

end

== matlab function model/IMU/Subsystem/Test Message Receiving ==
  data: msg input
function fcn(msg)
    disp(msg.Orientation.X);
    disp(msg.AngularVelocity.Y);
    disp(msg.LinearAcceleration.Z);
end
